simulink model "pratica4"  (R2021b)
settings: Solver=VariableStepAuto  StartTime=0.0  StopTime=24.00  RelTol=1e-3
values from neighbouring files (symbols this model uses):
  R = 1.15    [sel0620_lab4.m]
  T0 = (2*pi)/ws    [sel0620_lab4.m]
undefined symbols (not defined in the file or in its folder): den, num
settings Model: Creator=carlo  LastModifiedBy=carlo

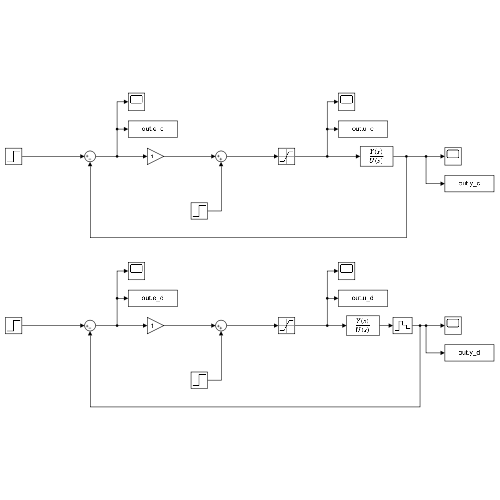
[thumbnail: Simulink's stored preview of the top-level diagram]
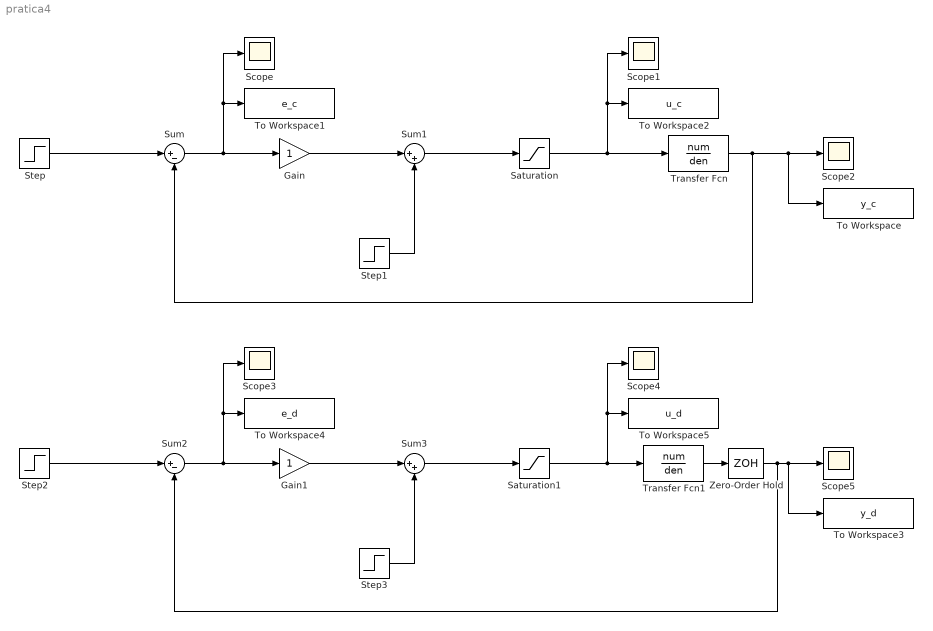
== system pratica4 ==
  Gain : Gain
  Gain1 : Gain
  Saturation : Saturate  UpperLimit=10  LowerLimit=-10
  Saturation1 : Saturate  UpperLimit=10  LowerLimit=-10
  Scope{,1..5} (6 alike) : Scope
  Step : Step  Time=0  After=R  SampleTime=0
  Step1 : Step  Time=12  After=0.26  SampleTime=0
  Step2 : Step  Time=0  After=R  SampleTime=0
  Step3 : Step  Time=12  After=0.26  SampleTime=0
  Sum : Sum  Inputs=|+-
  Sum1 : Sum  Inputs=|++
  Sum2 : Sum  Inputs=|+-
  Sum3 : Sum  Inputs=|++
  To Workspace : ToWorkspace  VariableName=y_c  SaveFormat=Timeseries  SampleTime=-1
  To Workspace1 : ToWorkspace  VariableName=e_c  SaveFormat=Timeseries  SampleTime=-1
  To Workspace2 : ToWorkspace  VariableName=u_c  SaveFormat=Timeseries  SampleTime=-1
  To Workspace3 : ToWorkspace  VariableName=y_d  SaveFormat=Timeseries  SampleTime=-1
  To Workspace4 : ToWorkspace  VariableName=e_d  SaveFormat=Timeseries  SampleTime=-1
  To Workspace5 : ToWorkspace  VariableName=u_d  SaveFormat=Timeseries  SampleTime=-1
  Transfer Fcn : TransferFcn  Numerator=num  Denominator=den
  Transfer Fcn1 : TransferFcn  Numerator=num  Denominator=den
  Zero-Order Hold : ZeroOrderHold  SampleTime=T0
  wires:
  Step/1 -> Sum/1
  Sum/1 -> To Workspace1/1, Scope/1, Gain/1
  Transfer Fcn/1 -> Sum/2, To Workspace/1, Scope2/1
  Saturation/1 -> To Workspace2/1, Scope1/1, Transfer Fcn/1
  Gain/1 -> Sum1/1
  Sum1/1 -> Saturation/1
  Step1/1 -> Sum1/2
  Zero-Order Hold/1 -> Sum2/2, To Workspace3/1, Scope5/1
  Step3/1 -> Sum3/2
  Saturation1/1 -> To Workspace5/1, Scope4/1, Transfer Fcn1/1
  Sum2/1 -> To Workspace4/1, Scope3/1, Gain1/1
  Gain1/1 -> Sum3/1
  Transfer Fcn1/1 -> Zero-Order Hold/1
  Step2/1 -> Sum2/1
  Sum3/1 -> Saturation1/1
